simulink model "conversion"  (R2021b)
settings: Solver=VariableStepAuto  StartTime=0.0  StopTime=10.0  RelTol=1e-3
values from neighbouring files (symbols this model uses):
  X_sim = test_raw(ii).X    [raw_converter.m]
  Xtare_raw = [870 1250 2036 2836 3410]    [callback.m]
  Xtare_real = [-127.5 -80 0 80 127.5] * 1e-3    [callback.m]
  Y_sim = test_raw(ii).Y    [raw_converter.m]
  Ytare_raw = [890 1370 2040 2690 3409]    [callback.m]
  Ytare_real = [-97.5 -50 0 50 110]*1e-3    [callback.m]
settings Model: Creator=ernesto  LastModifiedBy=ernesto

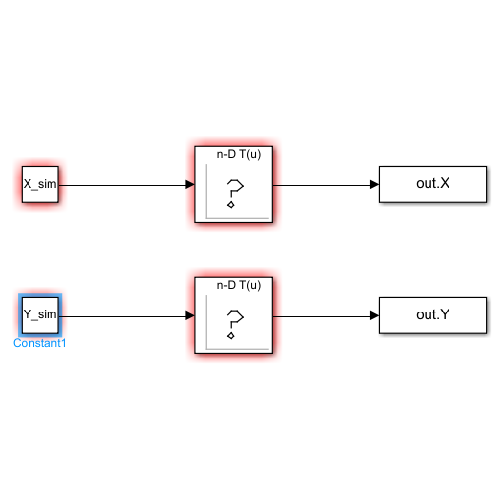
[thumbnail: Simulink's stored preview of the top-level diagram]
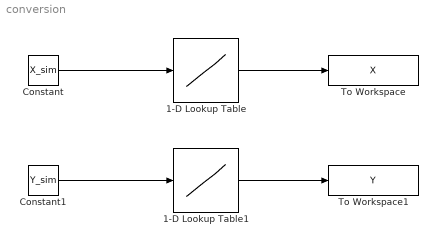
== system conversion ==
  1-D Lookup Table : Lookup_n-D  NumberOfTableDimensions=1  BreakpointsForDimension1=Xtare_raw  Table=Xtare_real  InternalRulePriority=Speed  RndMeth=Simplest  InputSameDT=on
  1-D Lookup Table1 : Lookup_n-D  NumberOfTableDimensions=1  BreakpointsForDimension1=Ytare_raw  Table=Ytare_real  InternalRulePriority=Speed  RndMeth=Simplest  InputSameDT=on
  Constant : Constant  Value=X_sim
  Constant1 : Constant  Value=Y_sim
  To Workspace : ToWorkspace  VariableName=X  SaveFormat=Timeseries  SampleTime=-1
  To Workspace1 : ToWorkspace  VariableName=Y  SaveFormat=Timeseries  SampleTime=-1
  wires:
  Constant/1 -> 1-D Lookup Table/1
  1-D Lookup Table/1 -> To Workspace/1
  Constant1/1 -> 1-D Lookup Table1/1
  1-D Lookup Table1/1 -> To Workspace1/1
